simulink model "oil_fuel_model"  (R2026a)
settings: Solver=VariableStepAuto  StopTime=300
undefined symbols (not defined in the file): engine
settings Model: Creator=GOD  LastModifiedBy=GOD

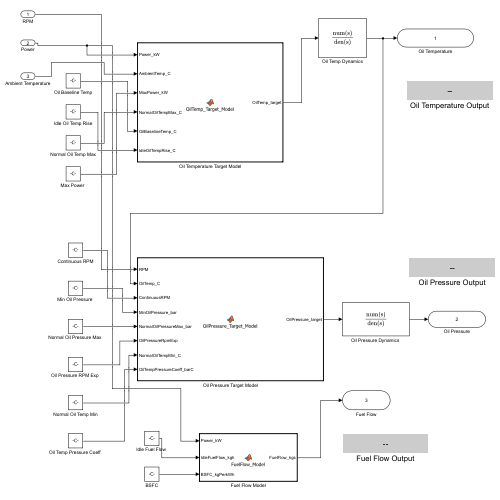
[thumbnail: Simulink's stored preview of the top-level diagram]
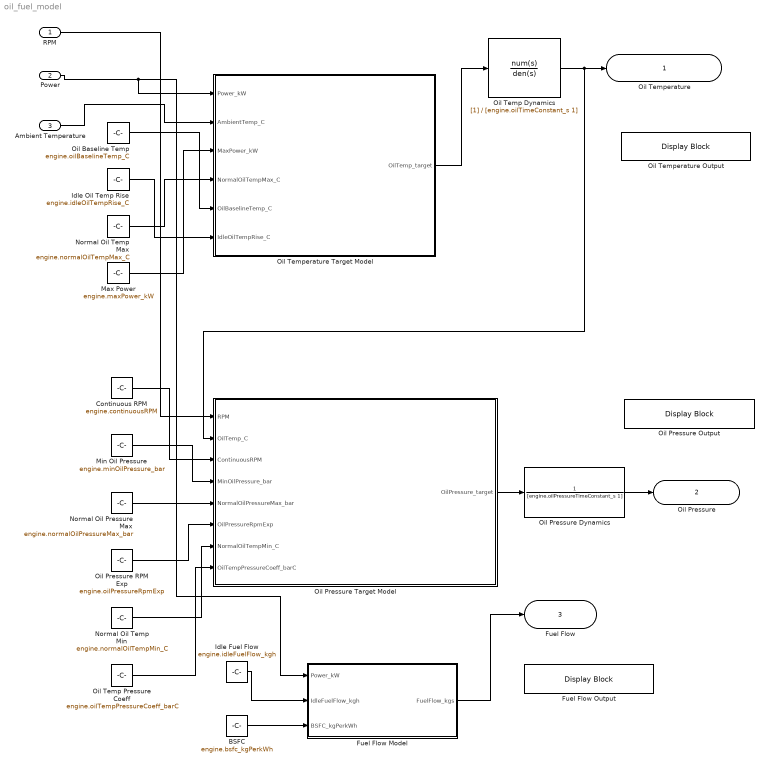
== system oil_fuel_model ==
  RPM : Inport
  Power : Inport  Port=2
  Ambient Temperature : Inport  Port=3
  BSFC : Constant  Value=engine.bsfc_kgPerkWh
  Continuous RPM : Constant  Value=engine.continuousRPM
  Fuel Flow Model : MATLAB Function  TreatAsAtomicUnit=on
  Fuel Flow Output : DisplayBlock  LabelPosition=Hide  Transparency=1  GridColor=[0.502, 0.502, 0.502]
  "Idle Fuel Flow " : Constant  Value=engine.idleFuelFlow_kgh
  Idle Oil Temp Rise : Constant  Value=engine.idleOilTempRise_C
  "Max Power " : Constant  Value=engine.maxPower_kW
  "Min Oil Pressure " : Constant  Value=engine.minOilPressure_bar
  "Normal Oil Pressure Max " : Constant  Value=engine.normalOilPressureMax_bar
  Normal Oil Temp Max : Constant  Value=engine.normalOilTempMax_C
  Normal Oil Temp Min : Constant  Value=engine.normalOilTempMin_C
  Oil Baseline Temp : Constant  Value=engine.oilBaselineTemp_C
  "Oil Pressure Dynamics " : TransferFcn  Denominator=[engine.oilPressureTimeConstant_s 1]
  Oil Pressure Output : DisplayBlock  LabelPosition=Hide  Transparency=1  GridColor=[0.502, 0.502, 0.502]
  "Oil Pressure RPM Exp " : Constant  Value=engine.oilPressureRpmExp
  Oil Pressure Target Model : MATLAB Function  TreatAsAtomicUnit=on
  Oil Temp Dynamics : TransferFcn  Denominator=[engine.oilTimeConstant_s 1]
  "Oil Temp Pressure Coeff " : Constant  Value=engine.oilTempPressureCoeff_barC
  Oil Temperature Output : DisplayBlock  LabelPosition=Hide  Transparency=1  GridColor=[0.502, 0.502, 0.502]
  Oil Temperature Target Model : MATLAB Function  TreatAsAtomicUnit=on
  Oil Temperature : Outport
  Oil Pressure : Outport  Port=2
  Fuel Flow : Outport  Port=3
  wires:
  "Max Power "/1 -> Oil Temperature Target Model/3(MaxPower_kW)
  Normal Oil Temp Max/1 -> Oil Temperature Target Model/4(NormalOilTempMax_C)
  Idle Oil Temp Rise/1 -> Oil Temperature Target Model/6(IdleOilTempRise_C)
  Oil Baseline Temp/1 -> Oil Temperature Target Model/5(OilBaselineTemp_C)
  Oil Temperature Target Model/1(OilTemp_target) -> Oil Temp Dynamics/1
  Continuous RPM/1 -> Oil Pressure Target Model/3(ContinuousRPM)
  "Min Oil Pressure "/1 -> Oil Pressure Target Model/4(MinOilPressure_bar)
  "Normal Oil Pressure Max "/1 -> Oil Pressure Target Model/5(NormalOilPressureMax_bar)
  "Oil Pressure RPM Exp "/1 -> Oil Pressure Target Model/6(OilPressureRpmExp)
  Normal Oil Temp Min/1 -> Oil Pressure Target Model/7(NormalOilTempMin_C)
  "Oil Temp Pressure Coeff "/1 -> Oil Pressure Target Model/8(OilTempPressureCoeff_barC)
  Oil Pressure Target Model/1(OilPressure_target) -> "Oil Pressure Dynamics "/1
  "Oil Pressure Dynamics "/1 -> Oil Pressure/1
  Oil Temp Dynamics/1 -> Oil Pressure Target Model/2(OilTemp_C), Oil Temperature/1
  "Idle Fuel Flow "/1 -> Fuel Flow Model/2(IdleFuelFlow_kgh)
  BSFC/1 -> Fuel Flow Model/3(BSFC_kgPerkWh)
  Fuel Flow Model/1(FuelFlow_kgs) -> Fuel Flow/1
  Ambient Temperature/1 -> Oil Temperature Target Model/2(AmbientTemp_C)
  RPM/1 -> Oil Pressure Target Model/1(RPM)
  Power/1 -> Fuel Flow Model/1(Power_kW), Oil Temperature Target Model/1(Power_kW)

== matlab function oil_fuel_model/Oil Pressure Target Model ==
  data: RPM input; OilPressure_target output; OilTemp_C input; ContinuousRPM input; MinOilPressure_bar input; NormalOilPressureMax_bar input; OilPressureRpmExp input; NormalOilTempMin_C input; OilTempPressureCoeff_barC input
function OilPressure_target = OilPressure_Target_Model(RPM, OilTemp_C, ...
                                    ContinuousRPM, MinOilPressure_bar, ...
                                    NormalOilPressureMax_bar, OilPressureRpmExp, ...
                                    NormalOilTempMin_C, OilTempPressureCoeff_barC)
% Engineering-assumption steady-state oil pressure target.
% Pressure rises with RPM (oil pump is engine-driven) and falls as
% oil gets hotter/thinner than its normal operating range.
rpmFraction = RPM / ContinuousRPM;
if rpmFraction < 0
    rpmFraction = 0;
elseif rpmFraction > 1
    rpmFraction = 1;
end

pressureFromRPM = MinOilPressure_bar + (NormalOilPressureMax_bar - MinOilPressure_bar) * rpmFraction^OilPressureRpmExp;

tempExcess = OilTemp_C - NormalOilTempMin_C;
if tempExcess < 0
    tempExcess = 0;
end
tempDrop = OilTempPressureCoeff_barC * tempExcess;

OilPressure_target = pressureFromRPM - tempDrop;
if OilPressure_target < 0
    OilPressure_target = 0;
end
end

== matlab function oil_fuel_model/Oil Temperature Target Model ==
  data: Power_kW input; OilTemp_target output; AmbientTemp_C input; MaxPower_kW input; NormalOilTempMax_C input; OilBaselineTemp_C input; IdleOilTempRise_C input
function OilTemp_target = OilTemp_Target_Model(Power_kW, AmbientTemp_C, ...
                                    MaxPower_kW, NormalOilTempMax_C, ...
                                    OilBaselineTemp_C, IdleOilTempRise_C)
% Engineering-assumption steady-state oil temperature target.
% Oil heats up with engine power output, starting from a baseline
% idle temperature above ambient.
powerFraction = Power_kW / MaxPower_kW;
if powerFraction < 0
    powerFraction = 0;
elseif powerFraction > 1
    powerFraction = 1;
end

OilTemp_target = AmbientTemp_C + IdleOilTempRise_C + ...
    (NormalOilTempMax_C - OilBaselineTemp_C - IdleOilTempRise_C) * powerFraction;
end

== matlab function oil_fuel_model/Fuel Flow Model ==
  data: Power_kW input; FuelFlow_kgs output; IdleFuelFlow_kgh input; BSFC_kgPerkWh input
function FuelFlow_kgs = FuelFlow_Model(Power_kW, IdleFuelFlow_kgh, BSFC_kgPerkWh)
% Engineering-assumption fuel flow model.
% Fuel flow is a baseline idle flow plus a rate proportional to power
% output (brake-specific fuel consumption). Fuel flow is treated as
% instantaneous -- no thermal lag, unlike CHT/EGT/OilTemp.
if Power_kW < 0
    Power_kW = 0;
end

FuelFlow_kgh = IdleFuelFlow_kgh + BSFC_kgPerkWh * Power_kW;
FuelFlow_kgs = FuelFlow_kgh / 3600;
end
